simulink model "APS"  (R2021a)
settings: Solver=FixedStepAuto  StartTime=0.0  StopTime=10  FixedStep=0.2  RelTol=1e-3
values from neighbouring files (symbols this model uses):
  K_steer = 57.29578    [Parameter.m]
  K_trains = 17.43769628    [Parameter.m]
  Rmin = 5    [Parameter.m]    (also in main.m = 6)
  Ts = 0.2    [Parameter.m]
  v0 = 1    [Parameter.m]
libraries: simulink x4
settings Model: Creator=6000022764  LastModifiedBy=6000022764

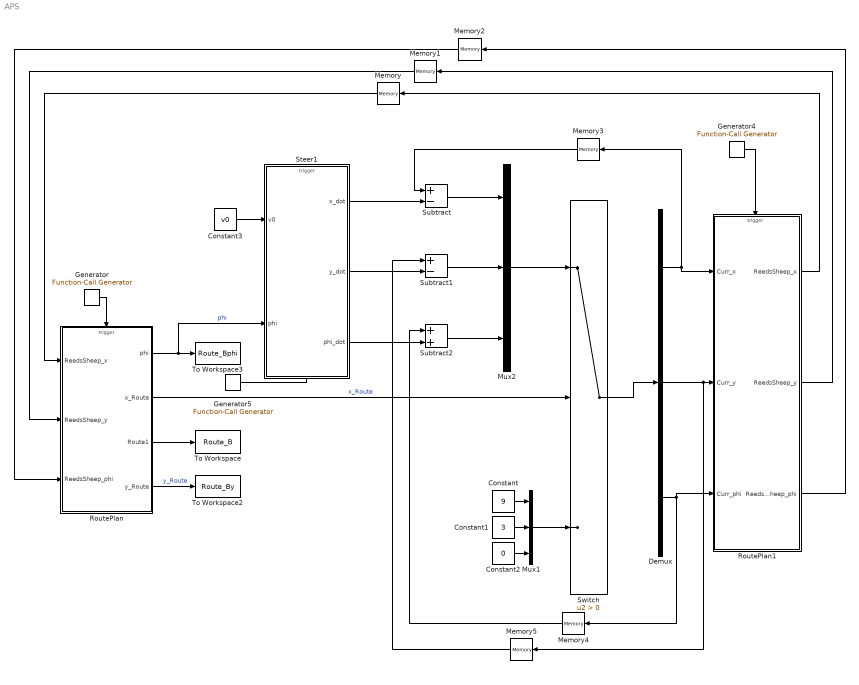
== system APS ==
  Constant : Constant  Value=9
  Constant1 : Constant  Value=3
  Constant2 : Constant  Value=0
  Constant3 : Constant  Value=v0
  Demux : Demux  Outputs=3
  Generator : simulink/Ports & Subsystems/Function-Call Generator  sample_time=0.2  numberOfIterations=1  DisallowWideOutput=off
      settings: AttributesFormatString=sample_time = %<sample_time>
  Generator4 : simulink/Ports & Subsystems/Function-Call Generator  sample_time=0.2  numberOfIterations=1  DisallowWideOutput=off
      settings: AttributesFormatString=sample_time = %<sample_time>
  Generator5 : simulink/Ports & Subsystems/Function-Call Generator  sample_time=0.2  numberOfIterations=1  DisallowWideOutput=off
      settings: AttributesFormatString=sample_time = %<sample_time>
  Memory{,1..2,4} (4 alike) : Memory
  Memory3 : Memory  InitialCondition=9
  Memory5 : Memory  InitialCondition=3
  Mux1 : Mux  Inputs=3
  Mux2 : Mux  Inputs=3
  RoutePlan : Subsystem  Description=B样条曲线
      settings: AttributesFormatString=%<Description>
  RoutePlan1 : Subsystem  Description=ReedsSheep曲线
      settings: AttributesFormatString=%<Description>
  Steer1 : Subsystem  Description=车辆运动学模型
      settings: AttributesFormatString=%<Description>
  Subtract : Sum  Inputs=+-
  Subtract1 : Sum  Inputs=+-
  Subtract2 : Sum
  Switch : Switch  Criteria=u2 > Threshold
  To Workspace : ToWorkspace  VariableName=Route_B  SampleTime=-1
  To Workspace2 : ToWorkspace  VariableName=Route_By  SampleTime=-1
  To Workspace3 : ToWorkspace  VariableName=Route_Bphi  SampleTime=-1
  wires:
  Generator4/1 -> RoutePlan1/Trigger
  Generator/1 -> RoutePlan/Trigger
  RoutePlan/3(Route1) -> To Workspace/1
  RoutePlan1/1(ReedsSheep_x) -> Memory/1
  RoutePlan1/2(ReedsSheep_y) -> Memory1/1
  RoutePlan1/3(ReedsSheep_phi) -> Memory2/1
  Memory/1 -> RoutePlan/1(ReedsSheep_x)
  Memory1/1 -> RoutePlan/2(ReedsSheep_y)
  Memory2/1 -> RoutePlan/3(ReedsSheep_phi)
  RoutePlan/1(phi) -> To Workspace3/1, Steer1/2(phi)  "phi"
  RoutePlan/2(x_Route) -> Switch/2  "x_Route"
  Demux/1 -> Memory3/1, RoutePlan1/1(Curr_x)
  Demux/2 -> Memory5/1, RoutePlan1/2(Curr_y)
  Demux/3 -> RoutePlan1/3(Curr_phi), Memory4/1
  Switch/1 -> Demux/1
  Constant/1 -> Mux1/1
  Constant1/1 -> Mux1/2
  Constant2/1 -> Mux1/3
  Mux1/1 -> Switch/3
  Constant3/1 -> Steer1/1(v0)
  Steer1/1(x_dot) -> Subtract/2
  Steer1/3(phi_dot) -> Subtract2/2
  Steer1/2(y_dot) -> Subtract1/2
  Subtract/1 -> Mux2/1
  Subtract1/1 -> Mux2/2
  Subtract2/1 -> Mux2/3
  RoutePlan/4(y_Route) -> To Workspace2/1  "y_Route"
  Mux2/1 -> Switch/1
  Generator5/1 -> Steer1/Trigger
  Memory3/1 -> Subtract/1
  Memory4/1 -> Subtract2/1
  Memory5/1 -> Subtract1/1

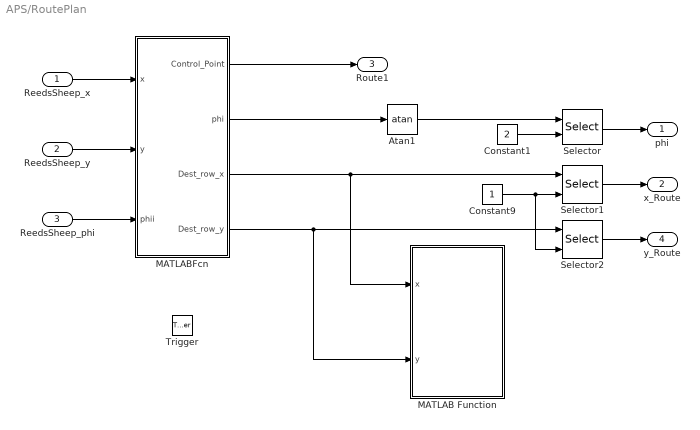
== system APS/RoutePlan ==
  ReedsSheep_x : Inport
  ReedsSheep_y : Inport  Port=2
  ReedsSheep_phi : Inport  Port=3
  Trigger : TriggerPort  TriggerType=function-call  VariantControl=Variant  PortDimensions=1
  Atan1 : Trigonometry  Operator=atan
  Constant1 : Constant  Value=2
  Constant9 : Constant
  MATLAB Function : MATLAB Function  TreatAsAtomicUnit=on
  MATLABFcn : MATLAB Function  Description=5次B样条开Clamped  TreatAsAtomicUnit=on
      settings: AttributesFormatString=%<Description>
  Selector : Selector  InputPortWidth=501  IndexOptions=Index vector (port)  Indices=1  OutputSizes=1
      settings: AttributesFormatString=size = %<InputPortWidth>
  Selector1 : Selector  InputPortWidth=501  IndexOptions=Index vector (port)  Indices=1  OutputSizes=1
      settings: AttributesFormatString=size = %<InputPortWidth>
  Selector2 : Selector  InputPortWidth=501  IndexOptions=Index vector (port)  Indices=1  OutputSizes=1
      settings: AttributesFormatString=size = %<InputPortWidth>
  phi : Outport  InitialOutput=0
  x_Route : Outport  Port=2  InitialOutput=9
  Route1 : Outport  Port=3
  y_Route : Outport  Port=4  InitialOutput=3
  wires:
  MATLABFcn/1(Control_Point) -> Route1/1
  MATLABFcn/2(phi) -> Atan1/1
  Selector/1 -> phi/1
  Constant9/1 -> Selector2/2, Selector1/2
  Atan1/1 -> Selector/1
  MATLABFcn/3(Dest_row_x) -> MATLAB Function/1(x), Selector1/1
  Selector1/1 -> x_Route/1
  Selector2/1 -> y_Route/1
  MATLABFcn/4(Dest_row_y) -> MATLAB Function/2(y), Selector2/1
  ReedsSheep_x/1 -> MATLABFcn/1(x)
  ReedsSheep_y/1 -> MATLABFcn/2(y)
  ReedsSheep_phi/1 -> MATLABFcn/3(phii)
  Constant1/1 -> Selector/2

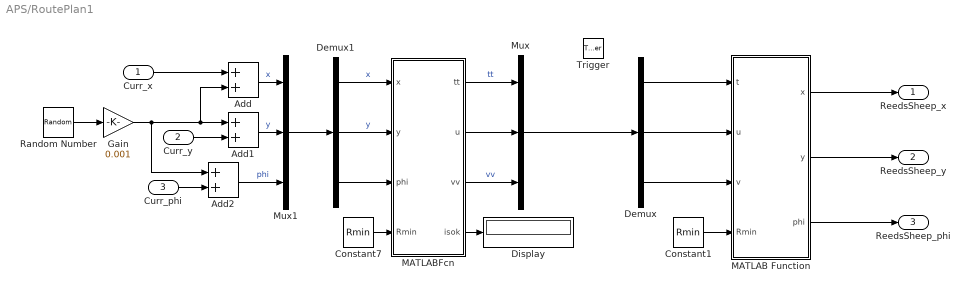
== system APS/RoutePlan1 ==
  Curr_x : Inport
  Curr_y : Inport  Port=2
  Curr_phi : Inport  Port=3
  Trigger : TriggerPort  TriggerType=function-call  VariantControl=Variant  PortDimensions=1
  Add : Sum
  Add1 : Sum
  Add2 : Sum
  Constant1 : Constant  Value=Rmin
  Constant7 : Constant  Value=Rmin
  Demux : Demux  Outputs=3
  Demux1 : Demux  Outputs=3
  Display : Display
  Gain : Gain  Gain=0.001
  MATLAB Function : MATLAB Function  TreatAsAtomicUnit=on
  MATLABFcn : MATLAB Function  Description=LSR  TreatAsAtomicUnit=on
      settings: AttributesFormatString=%<Description>
  Mux : Mux  Inputs=3
  Mux1 : Mux  Inputs=3
  Random Number : RandomNumber
  ReedsSheep_x : Outport
  ReedsSheep_y : Outport  Port=2
  ReedsSheep_phi : Outport  Port=3
  wires:
  Gain/1 -> Add2/1, Add/2, Add1/1
  Curr_x/1 -> Add/1
  Curr_y/1 -> Add1/2
  Curr_phi/1 -> Add2/2
  Constant7/1 -> MATLABFcn/4(Rmin)
  Constant1/1 -> MATLAB Function/4(Rmin)
  MATLABFcn/2(u) -> Mux/2
  MATLABFcn/1(tt) -> Mux/1  "tt"
  MATLABFcn/3(vv) -> Mux/3  "vv"
  Demux/2 -> MATLAB Function/2(u)
  Demux/1 -> MATLAB Function/1(t)
  Demux/3 -> MATLAB Function/3(v)
  Add/1 -> Mux1/1  "x"
  Add1/1 -> Mux1/2  "y"
  Add2/1 -> Mux1/3  "phi"
  Demux1/2 -> MATLABFcn/2(y)  "y"
  Demux1/1 -> MATLABFcn/1(x)  "x"
  Demux1/3 -> MATLABFcn/3(phi)
  Mux1/1 -> Demux1/1
  Random Number/1 -> Gain/1
  MATLAB Function/1(x) -> ReedsSheep_x/1
  MATLAB Function/2(y) -> ReedsSheep_y/1
  MATLAB Function/3(phi) -> ReedsSheep_phi/1
  Mux/1 -> Demux/1
  MATLABFcn/4(isok) -> Display/1

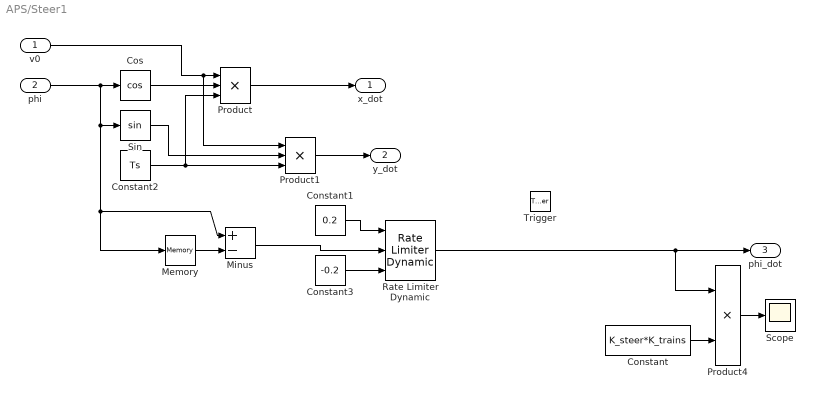
== system APS/Steer1 ==
  v0 : Inport
  phi : Inport  Port=2
  Trigger : TriggerPort  TriggerType=function-call  VariantControl=Variant  PortDimensions=1
  Constant : Constant  Value=K_steer*K_trains
  Constant1 : Constant  Value=0.2
  Constant2 : Constant  Value=Ts
  Constant3 : Constant  Value=-0.2
  Cos : Trigonometry  Operator=cos
  Memory : Memory  InheritSampleTime=on
  Minus : Sum  Inputs=+-
  Product : Product  Inputs=3  LockScale=on
  Product1 : Product  Inputs=3  LockScale=on
  Product4 : Product  LockScale=on
  Rate Limiter Dynamic : simulink/Discontinuities/Rate Limiter Dynamic
  Scope : Scope
  Sin : Trigonometry
  x_dot : Outport  InitialOutput=0
  y_dot : Outport  Port=2  InitialOutput=0
  phi_dot : Outport  Port=3  InitialOutput=0
  wires:
  Product4/1 -> Scope/1
  Constant/1 -> Product4/2
  Sin/1 -> Product1/2
  v0/1 -> Product/1, Product1/1
  Constant2/1 -> Product/3, Product1/3
  Product1/1 -> y_dot/1
  Cos/1 -> Product/2
  phi/1 -> Cos/1, Minus/1, Memory/1, Sin/1
  Product/1 -> x_dot/1
  Rate Limiter Dynamic/1 -> Product4/1, phi_dot/1
  Constant1/1 -> Rate Limiter Dynamic/1
  Constant3/1 -> Rate Limiter Dynamic/3
  Memory/1 -> Minus/2
  Minus/1 -> Rate Limiter Dynamic/2

== matlab function APS/RoutePlan1/MATLAB Function ==
  data: t input; u input; v input; Rmin input; x output; y output; phi output
function [x,y,phi] = fcn(t,u,v,Rmin)
l = 2.648; %轴距 m
L = 4.586; %车长 m
Lw = 1.522; %轮距
W = 1.772; %车宽
if t<=0
    t =0.01;
end
xxx  = zeros(1,5);
yyy  = zeros(1,5);
phiphiphi = zeros(1,5);
Numtt = 1;Numvv =1;
for theta = [0 t/4 t/2 t*3/4 t]
    
    xxx(Numtt) = Rmin*sin(theta);
    yyy(Numtt) = Rmin*(1-cos(theta));
    phiphiphi(Numtt) = theta;
    Numtt = Numtt+1;
end
xxu = [Rmin*sin(t)+u*cos(t)/5 Rmin*sin(t)+2*u*cos(t)/5 Rmin*sin(t)+u*cos(t)*3/5 Rmin*sin(t)+u*cos(t)*4/5];
yyu = [Rmin*(1-cos(t))+u*sin(t)/5 Rmin*(1-cos(t))+2*u*sin(t)/5 Rmin*(1-cos(t))+3*u*sin(t)/5 Rmin*(1-cos(t))+4*u*sin(t)/5];
if v > 0
    xx = zeros(1,6);
    yy = zeros(1,6);
    phiphi = zeros(1,6);
    for theta = [t t-v/5 t-v*2/5 t-v*3/5 t-v*4/5 t-v]
        xx(Numvv) = u * cos(t)-Rmin*(sin(theta)-2*sin(t));
        yy(Numvv) = u * sin(t)+Rmin*(cos(theta)-2*cos(t)+1);
        phiphi(Numvv) = theta;
        Numvv = Numvv+1;
    end
    % plot(x,y);
    
    % 前轴中心点坐标fw
    xfw = xx(end) + l*cos(t-v);
    yfw = yy(end) + l*sin(t-v);
    % 后轴中心点坐标rw
    xrw = xx(end);
    yrw = yy(end) ;
    % 车辆四轮与地面交点
    xa = xx(end)  + Lw*sin(t-v)/2; % 右后轮与地面交点坐标
    ya = yy(end)  - Lw*cos(t-v)/2;
    xb = xx(end) + l*cos(t-v) + Lw*sin(t-v)/2; % 右前轮与地面交点坐标
    yb = yy(end) + l*sin(t-v) - Lw*cos(t-v)/2;
    xc = xx(end) + l*cos(t-v) - Lw*sin(t-v)/2; % 左前轮与地面交点坐标
    yc = yy(end) + l*sin(t-v) + Lw*cos(t-v)/2;
    xd = xx(end)  - Lw*sin(t-v)/2; % 左后轮与地面交点坐标
    yd = yy(end)  + Lw*cos(t-v)/2;
    % 车身四个顶点坐标
    XA = xx(end) +l*cos(t-v)/2 - L*cos(t-v)/2 + W*sin(t-v)/2; % 车辆右后顶点
    YA = yy(end) + l*sin(t-v)/2- L*sin(t-v)/2 - W*cos(t-v)/2;
    XB = xx(end) +l*cos(t-v)/2 + L*cos(t-v)/2 + W*sin(t-v)/2; % 车辆右前顶点
    YB = yy(end) + l*sin(t-v)/2+ L*sin(t-v)/2 - W*cos(t-v)/2;
    XC = xx(end) +l*cos(t-v)/2 + L*cos(t-v)/2 - W*sin(t-v)/2; % 车辆左前顶点
    YC = yy(end) + l*sin(t-v)/2+ L*sin(t-v)/2 + W*cos(t-v)/2;
    XD = xx(end) +l*cos(t-v)/2 - L*cos(t-v)/2 - W*sin(t-v)/2; % 车辆左后顶点
    YD = yy(end) + l*sin(t-v)/2- L*sin(t-v)/2 + W*cos(t-v)/2;
else
    xx = [xxx(end) u*cos(t)/5+xxx(end) u*cos(t)*2/5+xxx(end) u*cos(t)*3/5+xxx(end) u*cos(t)*4/5+xxx(end) u*cos(t)+xxx(end)];
    yy = [yyy(end) u*sin(t)/5+yyy(end) u*sin(t)*2/5+yyy(end) u*sin(t)*3/5+yyy(end) u*sin(t)*4/5+yyy(end) u*sin(t)+yyy(end)];
    phiphi = [t t t t t t];
    % 前轴中心点坐标fw
    xfw = xx(end) + l*cos(t);
    yfw = yy(end) + l*sin(t);
    % 后轴中心点坐标rw
    xrw = xx(end);
    yrw = yy(end);
    % 车辆四轮与地面交点
    xa = xx(end)  + Lw*sin(t)/2; % 右后轮与地面交点坐标
    ya = yy(end)  - Lw*cos(t)/2;
    xb = xx(end) + l*cos(t) + Lw*sin(t)/2; % 右前轮与地面交点坐标
    yb = yy(end) + l*sin(t) - Lw*cos(t)/2;
    xc = xx(end) + l*cos(t) - Lw*sin(t)/2; % 左前轮与地面交点坐标
    yc = yy(end) + l*sin(t) + Lw*cos(t)/2;
    xd = xx(end)  - Lw*sin(t)/2; % 左后轮与地面交点坐标
    yd = yy(end)  + Lw*cos(t)/2;
    % 车身四个顶点坐标
    XA = xx(end) +l*cos(t)/2- L*cos(t)/2 + W*sin(t)/2; % 车辆右后顶点
    YA = yy(end) +l*sin(t)/2- L*sin(t)/2 - W*cos(t)/2;
    XB = xx(end) +l*cos(t)/2+ L*cos(t)/2 + W*sin(t)/2; % 车辆右前顶点
    YB = yy(end) +l*sin(t)/2+ L*sin(t)/2 - W*cos(t)/2;
    XC = xx(end) +l*cos(t)/2+ L*cos(t)/2 - W*sin(t)/2; % 车辆左前顶点
    YC = yy(end) +l*sin(t)/2+ L*sin(t)/2 + W*cos(t)/2;
    XD = xx(end) +l*cos(t)/2- L*cos(t)/2 - W*sin(t)/2; % 车辆左后顶点
    YD = yy(end) +l*sin(t)/2- L*sin(t)/2 + W*cos(t)/2;
end

x = [xxx xxu xx];
y = [yyy yyu yy];
phi = [phiphiphi phiphi];

ABX = [XA XB];
ABY = [YA YB];
BCX = [XB XC];
BCY = [YB YC];
CDX = [XC XD];
CDY = [YC YD];
DAX = [XD XA];
DAY = [YD YA];
bcx = [xb xc];
bcy = [yb yc];
dax = [xd xa];
day = [yd ya];
frx = [xfw xrw];
fry = [yfw yrw];
slotx = [-5 -1 -1 6.5 6.5 15];
sloty = [1 1 -1.2 -1.2 1 1];
plot(x,y,slotx,sloty,ABX,ABY,BCX,BCY,CDX,CDY,DAX,DAY,bcx,bcy,dax,day,frx,fry,'Color','r');
hold off;
axis([-5 15 -2 6])

== matlab function APS/RoutePlan1/MATLABFcn ==
  data: tt output; u output; vv output; x input; isok output; y input; phi input; Rmin input
% formula 8.2
function [tt,u,vv,isok] = LpSpRp(x,y,phi,Rmin)
[t1,u1] = cart2pol(x+Rmin*sin(phi),y-Rmin*(1+cos(phi)));
if u1^2 >= 4*Rmin^2 % 判断LSR
    u = sqrt(u1^2-4*Rmin^2);
    theta = atan2(2*Rmin,u);
    tt = t1+theta;
    tt = rem(tt,2*pi);
    if tt < -pi
        tt = tt+2*pi;
    elseif tt > pi
        tt = tt-2*pi;
    end
    vv = tt-phi;
    vv = rem(vv,2*pi);
    if vv < -pi
        vv = vv+2*pi;
    elseif vv > pi
        vv = vv-2*pi;
    end
    if tt >= 0 && vv > 0 % 判断LSR
        isok = true;
        return
    else  % 判断不是LSR
        isok = false;
        vv =0;
        tt = phi;
        u = (x-Rmin*sin(phi))/cos(phi);
        return;
    end  
else  % 判断不是LSR
    isok = false;
    vv =0;
    u = (x-Rmin*sin(phi))/cos(phi);
    tt = phi;
    if u<0
        u=0;
    end
    return;
end

== matlab function APS/RoutePlan/MATLAB Function ==
  data: x input; y input
function PlotVehicle(x,y) % x,y 车辆中心点坐标，phi 车辆航向角（车辆前后中轴线与坐标系X方向夹角）
    
%     % 车辆参数
%     L = 4.586; %车长 m
%     l = 2.648; %轴距 m
%     Lw = 1.522; %轮距
%     W = 1.772; %车宽
%     
%     x = x+l*cos(phi)/2;
%     y = y+l*sin(phi)/2;
%     
%     % 前轴中心点坐标fw
%     xfw = x + l*cos(phi)/2;
%     yfw = y + l*sin(phi)/2;
%     % 后轴中心点坐标rw
%     xrw = x - l*cos(phi)/2;
%     yrw = y - l*sin(phi)/2;
%     % 车辆四轮与地面交点
%     xa = x - l*cos(phi)/2 + Lw*sin(phi)/2; % 右后轮与地面交点坐标
%     ya = y - l*sin(phi)/2 - Lw*cos(phi)/2;
%     xb = x + l*cos(phi)/2 + Lw*sin(phi)/2; % 右前轮与地面交点坐标
%     yb = y + l*sin(phi)/2 - Lw*cos(phi)/2;
%     xc = x + l*cos(phi)/2 - Lw*sin(phi)/2; % 左前轮与地面交点坐标
%     yc = y + l*sin(phi)/2 + Lw*cos(phi)/2;
%     xd = x - l*cos(phi)/2 - Lw*sin(phi)/2; % 左后轮与地面交点坐标
%     yd = y - l*sin(phi)/2 + Lw*cos(phi)/2;
%     % 车身四个顶点坐标
%     XA = x - L*cos(phi)/2 + W*sin(phi)/2; % 车辆右后顶点
%     YA = y - L*sin(phi)/2 - W*cos(phi)/2;
%     XB = x + L*cos(phi)/2 + W*sin(phi)/2; % 车辆右前顶点
%     YB = y + L*sin(phi)/2 - W*cos(phi)/2;
%     XC = x + L*cos(phi)/2 - W*sin(phi)/2; % 车辆左前顶点
%     YC = y + L*sin(phi)/2 + W*cos(phi)/2;
%     XD = x - L*cos(phi)/2 - W*sin(phi)/2; % 车辆左后顶点
%     YD = y - L*sin(phi)/2 + W*cos(phi)/2;
%     ABX = [XA XB];
%     ABY = [YA YB];
%     BCX = [XB XC];
%     BCY = [YB YC];
%     CDX = [XC XD];
%     CDY = [YC YD];
%     DAX = [XD XA];
%     DAY = [YD YA];
%     bcx = [xb xc];
%     bcy = [yb yc];
%     dax = [xd xa];
%     day = [yd ya];
%     frx = [xfw xrw];
%     fry = [yfw yrw];
    plot(x,y,'Color','k');hold on;%,'LineWidth',3
%     plot([-5 -1.5 -1.5 6 6 15],[1 1 -1.2 -1.2 1 1],'LineWidth',2,'Color','k');
%     plot([-5 -3 -3 4 4 15],[1 1 -2 -2 1 1]);
%     axis([-5 15 -5 8]);
end

== matlab function APS/RoutePlan/MATLABFcn ==
  data: Control_Point output; x input; phi output; Dest_row_x output; Dest_row_y output; y input; phii input
function [Control_Point,phi,Dest_row_x,Dest_row_y] = fcn(x,y,phii)
% n,线条控制点数；k，阶次数
n =15; k =5;
% n =7; k =5;
P_dest = zeros(2,n);
P_dest(1,:) = x;
P_dest(2,:) = y;
% NodeVector = linspace(0,1,n+k+1); % 从0到1，设置均匀B样条节点区间；
% NodeVector = [0,0,0,0,0,0,0.2,0.4,0.6,0.8,1,1,1,1,1,1];
% NodeVector = [0,0,0,0,0,0,0.5,1,1,1,1,1,1];
% NodeVector = [0,0,0,0,0,0,0.1,0.2,0.3,0.4,0.5,0.6,0.7,0.8,0.9,1,1,1,1,1,1];
NodeVector = [0,0,0,0,0,0,1,2,3,4,5,6,7,8,9,10,10,10,10,10,10];
% 当起始点和终止点的重复度为最高次数加1是，开B样条变为Clamped B样条，当起始点和终止点重合且重复度为p+1时为闭B样条曲线。
Nik = zeros(n+k, k+1);
plot(P_dest(1, 1:n), P_dest(2, 1:n),...
    'o','LineWidth',1,...
    'MarkerEdgeColor','k',...
    'MarkerFaceColor','g',...
    'MarkerSize',6);hold on;
line(P_dest(1, 1:n), P_dest(2, 1:n));hold on;
% axis([-2,10,-2,10]);
umin =0;umax = 10;delta_u = 0.02;
Num = floor((umax-umin)/delta_u)+1;
Dest = zeros(2,Num);
Control_Point = zeros(Num,3);
Dest_row_x = zeros(Num,1);
Dest_row_y = zeros(Num,1);
m=1;
phi = zeros(Num,1);
N_i_5 = zeros(n,1);
for u = umin : delta_u : umax
    for i5 = 1:n
        for i4 = i5:i5+1
            for i3 = i5:i5+2
                for i2 = i5:i5+3
                    for i1 = i5:i5+4
                        for i = i5:i5+5
                            if (u >= NodeVector(i)) && (u < NodeVector(i+1))
                                Nik(i,1) = 1.0;
                            else
                                Nik(i,1) = 0.0;
                            end
                        end
                        Length1 = NodeVector(i1+1) - NodeVector(i1);
                        Length2 = NodeVector(i1+2) - NodeVector(i1+1);      % 支撑区间的长度
                        if Length1 == 0.0       % 规定0/0 = 0
                            Length1 = 1.0;
                        end
                        if Length2 == 0.0
                            Length2 = 1.0;
                        end
                        Nik(i1,2) = (u - NodeVector(i1)) / Length1 * Nik(i1,1) ...
                            + (NodeVector(i1+2) - u) / Length2 * Nik(i1+1,1);
                    end
                    Length1 = NodeVector(i2+2) - NodeVector(i2);
                    Length2 = NodeVector(i2+3) - NodeVector(i2+1);      % 支撑区间的长度
                    if Length1 == 0.0       % 规定0/0 = 0
                        Length1 = 1.0;
                    end
                    if Length2 == 0.0
                        Length2 = 1.0;
                    end
                    Nik(i2,3) = (u - NodeVector(i2)) / Length1 * Nik(i2,2) ...
                        + (NodeVector(i2+3) - u) / Length2 * Nik(i2+1,2);
                end
                Length1 = NodeVector(i3+3) - NodeVector(i3);
                Length2 = NodeVector(i3+4) - NodeVector(i3+1);      % 支撑区间的长度
                if Length1 == 0.0       % 规定0/0 = 0
                    Length1 = 1.0;
                end
                if Length2 == 0.0
                    Length2 = 1.0;
                end
                Nik(i3,4) = (u - NodeVector(i3)) / Length1 * Nik(i3,3) ...
                    + (NodeVector(i3+4) - u) / Length2 * Nik(i3+1,3);
            end
            Length1 = NodeVector(i4+4) - NodeVector(i4);
            Length2 = NodeVector(i4+5) - NodeVector(i4+1);      % 支撑区间的长度
            if Length1 == 0.0       % 规定0/0 = 0
                Length1 = 1.0;
            end
            if Length2 == 0.0
                Length2 = 1.0;
            end
            Nik(i4,5) = (u - NodeVector(i4)) / Length1 * Nik(i4,4) ...
                + (NodeVector(i4+5) - u) / Length2 * Nik(i4+1,4);
        end
        Length1 = NodeVector(i5+5) - NodeVector(i5);
        Length2 = NodeVector(i5+6) - NodeVector(i5+1);      % 支撑区间的长度
        if Length1 == 0.0       % 规定0/0 = 0
            Length1 = 1.0;
        end
        if Length2 == 0.0
            Length2 = 1.0;
        end
        Nik(i5,6) = (u - NodeVector(i5)) / Length1 * Nik(i5,5) ...
            + (NodeVector(i5+6) - u) / Length2 * Nik(i5+1,5);
        N_i_5(i5,1) = Nik(i5,6);
    end
    p_u = P_dest * N_i_5;
    Dest(:,m) = p_u;
    Dest_row_x(m,1) = p_u(1,1);
    Dest_row_y(m,1) = p_u(2,1);
    if m>1 && min(Dest(:,m))>0
        phi(m,1) = (Dest(2,m-1) - Dest(2,m))/(Dest(1,m-1) - Dest(1,m));
    end
    Control_Point(m,:) = [Dest(:,m)' phi(m,1) ];
    m = m+1;
    
end
% phi(1,1) = phii(1,1);
phi(end,1) = phii(1,end);
Dest_row_x(end) = P_dest(1,end);
Dest_row_y(end) = P_dest(2,end);
Dest_row_x = flipud(Dest_row_x);
Dest_row_y = flipud(Dest_row_y);
phi = flipud(phi);
